simulink subsystem "CartesianToServoDegrees"  (R2019b)
settings: Solver=VariableStepAuto  StartTime=0.0  StopTime=10.0  RelTol=1e-3
settings Model: Creator=toons  LastModifiedBy=killidaen

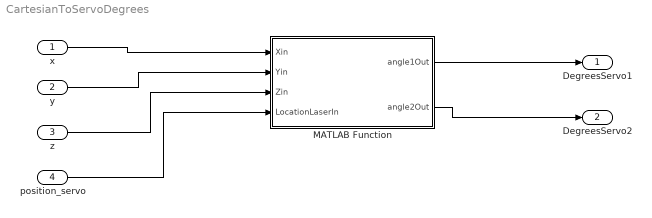
== system CartesianToServoDegrees ==
  x : Inport
  y : Inport  Port=2
  z : Inport  Port=3
  position_servo : Inport  Port=4
  MATLAB Function : MATLAB Function  TreatAsAtomicUnit=on
  DegreesServo1 : Outport
  DegreesServo2 : Outport  Port=2
  wires:
  x/1 -> MATLAB Function/1(Xin)
  y/1 -> MATLAB Function/2(Yin)
  z/1 -> MATLAB Function/3(Zin)
  position_servo/1 -> MATLAB Function/4(LocationLaserIn)
  MATLAB Function/1(angle1Out) -> DegreesServo1/1
  MATLAB Function/2(angle2Out) -> DegreesServo2/1

== matlab function CartesianToServoDegrees/MATLAB Function ==
  data: Xin input; angle1Out output; Yin input; Zin input; LocationLaserIn input; angle2Out output
function [angle1Out,angle2Out]= fcn(Xin,Yin,Zin,LocationLaserIn)

%tenzij verandering
lengthLaserPos = 0;

bestpos = [0,0,0];
bestpos(1) = Xin;
bestpos(2) = Yin;
bestpos(3) = Zin;
locationLaser = LocationLaserIn;


%calculate the first angle
  angle1 = atan2((bestpos(2) - locationLaser(2)),(bestpos(1) - locationLaser(1)));
  %update Laser location based on angle and the distance between joints
  updateLocationLaser = locationLaser;
  updateLocationLaser(1) = updateLocationLaser(1)+(lengthLaserPos*cos(angle1));
  updateLocationLaser(2) = updateLocationLaser(2)+(lengthLaserPos*sin(angle1));
  %calculate second angle based on musquitto and updated location
  angle2 = atan2(sqrt((bestpos(1) - updateLocationLaser(1)).^2 + (bestpos(2) - updateLocationLaser(2)).^2),((bestpos(3) - updateLocationLaser(3))));
  

  
  
angle1Out = angle1;
angle2Out = angle2;
